simulink model "Hinfinity_controller"  (R2025b)
settings: Solver=VariableStepAuto  StartTime=0.0  StopTime=15.0  RelTol=1e-8
undefined symbols (not defined in the file or in its folder): A, Ak, B, Bk, C, Ck, D, Dk, Ts
libraries: simulink x1
settings DataIOCC: SaveOutput=off  SignalLogging=off  DSMLogging=off  SaveTime=off  ReturnWorkspaceOutputs=off

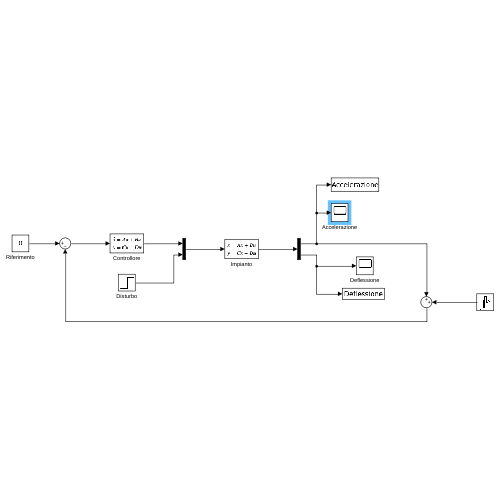
[thumbnail: Simulink's stored preview of the top-level diagram]
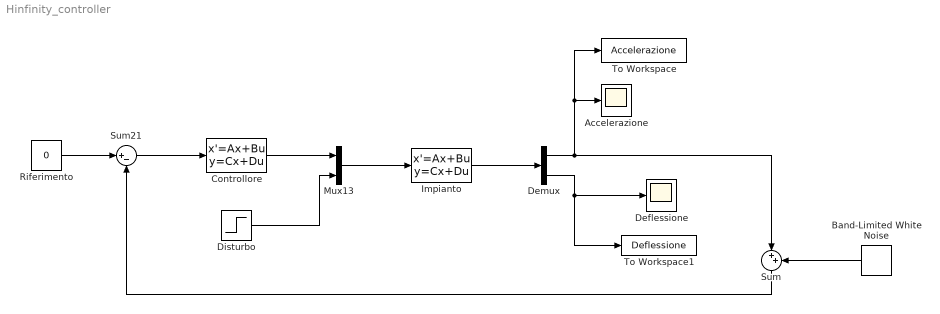
== system Hinfinity_controller ==
  Accelerazione : Scope
      settings: ActiveDisplayYMinimum=-0.576455439308971  ActiveDisplayYMaximum=0.89785519508276945
  Band-Limited White Noise : simulink/Sources/Band-Limited White Noise  Cov=1e-8  Ts=0.001  seed=[23341]
  Controllore : StateSpace  A=Ak  B=Bk  C=Ck  D=Dk  InitialCondition=0
  Deflessione : Scope
      settings: ActiveDisplayYMinimum=-1.6369929162069296E-6  ActiveDisplayYMaximum=1.4732936245862369E-5
  Demux : Demux  Outputs=2
  Disturbo : Step  Time=Ts  After=0.05  SampleTime=0
  Impianto : StateSpace  A=A  B=B  C=C  D=D  InitialCondition=0
  Mux13 : Mux  Inputs=2
  Riferimento : Constant  Value=0
  Sum : Sum  Inputs=|++
  Sum21 : Sum  Inputs=|+-
  To Workspace : ToWorkspace  VariableName=Accelerazione  SaveFormat=Timeseries  SampleTime=-1
  To Workspace1 : ToWorkspace  VariableName=Deflessione  SaveFormat=Timeseries  SampleTime=-1
  wires:
  Mux13/1 -> Impianto/1
  Sum21/1 -> Controllore/1
  Demux/1 -> Sum/1, To Workspace/1, Accelerazione/1
  Riferimento/1 -> Sum21/1
  Demux/2 -> To Workspace1/1, Deflessione/1
  Impianto/1 -> Demux/1
  Controllore/1 -> Mux13/1
  Disturbo/1 -> Mux13/2
  Sum/1 -> Sum21/2
  Band-Limited White Noise/1 -> Sum/2
